simulink model "task_1_scheme"  (R2024a)
settings: Solver=FixedStepAuto  StartTime=0.0  StopTime=60.0  FixedStep=0.001  RelTol=1e-3
settings Model: Creator=alexe  LastModifiedBy=alexe

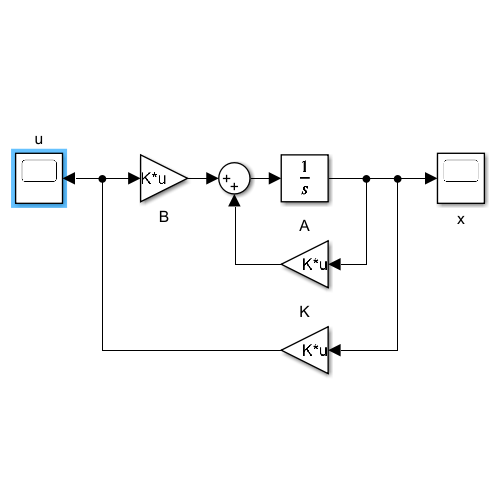
[thumbnail: Simulink's stored preview of the top-level diagram]
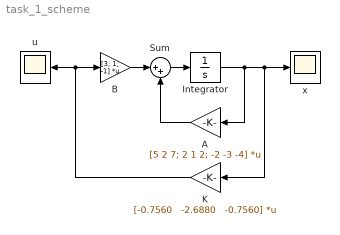
== system task_1_scheme ==
  A : Gain  Gain=[5 2 7; 2 1 2; -2 -3 -4]  Multiplication=Matrix(K*u)
  B : Gain  Gain=[3; 1; -1]  Multiplication=Matrix(K*u)
  Integrator : Integrator  InitialCondition=[1;1;1]
  K : Gain  Gain="[-0.7560   -2.6880   -0.7560]"  Multiplication=Matrix(K*u)
  Sum : Sum  Inputs=|++
  u : Scope
  x : Scope
  wires:
  B/1 -> Sum/1
  Sum/1 -> Integrator/1
  A/1 -> Sum/2
  Integrator/1 -> A/1, K/1, x/1
  K/1 -> B/1, u/1
